simulink model "rccg_digitalTwin"  (R2024a)
settings: Solver=VariableStepAuto  StartTime=0.0  StopTime=1  RelTol=1e-3
libraries: spsMultimeterLib x14, spsThreePhaseBreakerLib x9, spsThreePhaseSeriesRLCLoadLib x7, spsThreePhaseVIMeasurementLib x3, spsSynchronousMachinepuStandardLib x2, spsThreePhaseTransformerTwoWindingsLib x1, spsExcitationSystemLib x1, spsHydraulicTurbineandGovernorLib x1, spsThreePhaseParallelRLCLoadLib x1, sps_lib x1
settings Model: Creator=dogba  LastModifiedBy=dogba

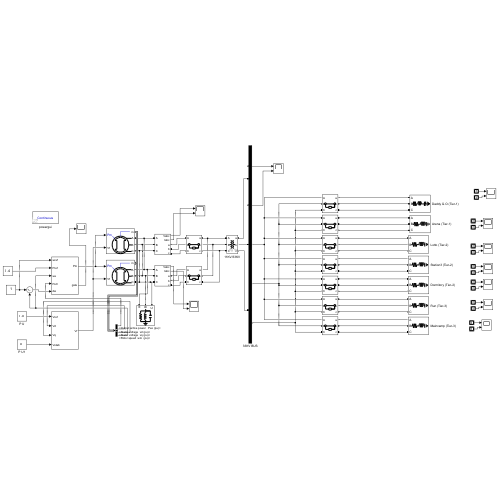
[thumbnail: Simulink's stored preview of the top-level diagram]
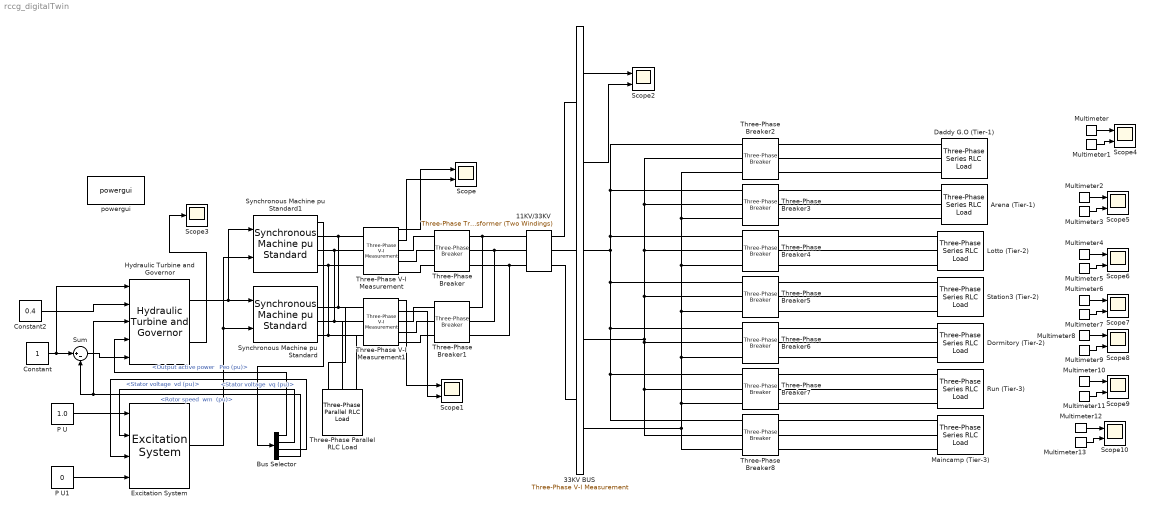
== system rccg_digitalTwin ==
  11KV/33KV : spsThreePhaseTransformerTwoWindingsLib/Three-Phase Transformer (Two Windings)  Winding1Connection=Yg  Winding2Connection=Yg  CoreType=Three single-phase transformers  SetSaturation=off  Hysteresis=off  DataFile='hysteresis'  SetInitialFlux=off  Measurements=None  UNITS=pu  NominalPower=[ 10e6 , 60 ]  Winding1=[ 11e3 , 0.002 , 0.08 ]  Winding2=[ 33e3 , 0.002 , 0.08 ]  Rm=500  Lm=500  L0=0.5  Saturation=[ 0,0 ; 0.0024,1.2 ; 1.0,1.52 ]  InitialFluxes=[ 0.8 , -0.8 , 0.7 ]  BreakLoop=off  DiscreteSolver=Trapezoidal iterative  DataType=off  TransfoNumber=1
  33KV BUS : spsThreePhaseVIMeasurementLib/Three-Phase V-I Measurement  VoltageMeasurement=phase-to-ground  SetLabelV=off  LabelV=Vabc  Vpu=off  VpuLL=off  CurrentMeasurement=yes  SetLabelI=off  LabelI=Iabc  Ipu=off  Pbase=100e6  Vbase=500e3  OutputType=Complex  PhasorSimulation=off  PSBequivalent=0
  Arena (Tier-1) : spsThreePhaseSeriesRLCLoadLib/Three-Phase Series RLC Load  LConnTagsString=A|B|C  Configuration=Y (grounded)  NominalVoltage=415  Vabc=[1e3 1e3 1e3]  Vabcp=[1e3 1e3 1e3]  NominalFrequency=50  UnbalancedPower=off  ActivePower=2e6  InductivePower=0.7e6  CapacitivePower=0  Pabc=[10e3 9e3 11e3]  QLabc=[100 90 110]  QCabc=[100 90 110]  Pabcp=[10e3 9e3 11e3]  QLabcp=[100 90 110]  QCabcp=[100 90 110]  Measurements=Branch voltages and currents  LoadType=constant PQ
  Bus Selector : BusSelector  OutputSignals="Output active power   Peo (pu),dq0 components.Stator voltage  vd (pu),dq0 components.Stator voltage  vq (pu),Mechanical.Rotor speed  wm  (pu)"
  Constant : Constant
  Constant2 : Constant  Value=0.4
  Daddy G.O (Tier-1) : spsThreePhaseSeriesRLCLoadLib/Three-Phase Series RLC Load  LConnTagsString=A|B|C  Configuration=Y (grounded)  NominalVoltage=415  Vabc=[1e3 1e3 1e3]  Vabcp=[1e3 1e3 1e3]  NominalFrequency=50  UnbalancedPower=off  ActivePower=1.5e6  InductivePower=0.4e6  CapacitivePower=100  Pabc=[10e3 9e3 11e3]  QLabc=[100 90 110]  QCabc=[100 90 110]  Pabcp=[10e3 9e3 11e3]  QLabcp=[100 90 110]  QCabcp=[100 90 110]  Measurements=Branch voltages and currents  LoadType=constant PQ
  Dormitory (Tier-2) : spsThreePhaseSeriesRLCLoadLib/Three-Phase Series RLC Load  LConnTagsString=A|B|C  Configuration=Y (grounded)  NominalVoltage=400  Vabc=[1e3 1e3 1e3]  Vabcp=[1e3 1e3 1e3]  NominalFrequency=50  UnbalancedPower=off  ActivePower=0.5e6  InductivePower=0.15e6  CapacitivePower=0  Pabc=[10e3 9e3 11e3]  QLabc=[100 90 110]  QCabc=[100 90 110]  Pabcp=[10e3 9e3 11e3]  QLabcp=[100 90 110]  QCabcp=[100 90 110]  Measurements=Branch voltages and currents  LoadType=constant PQ
  Excitation System : spsExcitationSystemLib/Excitation System  tr=20e-3  reg=[ 300, 0.001 ]  exc=[ 1, 0 ]  tgr=[ 0, 0 ]  damp=[ 0.001, 0.1 ]  sat=[ 0, 0 ]  lim=[ -11.5, 11.5, 0 ]  v0="[1.0  1.28]"
      settings: LibrarySourceBlock=sps_lib/Electrical Machines/Synchronous Machine Control/Excitation System
  Hydraulic Turbine and Governor : spsHydraulicTurbineandGovernorLib/Hydraulic Turbine and Governor  sm="[ 10/3  0.07 ]"  gate="[  0.01  0.97518  -0.1  0.1 ]"  reg="[  0.05  1.163  0.105  0  0.01  ]"  hyd="[  0  2.67  ]"  dref=0  po=0.7516
      settings: LibrarySourceBlock=|
      | sps_lib/Electrical Machines/Synchronous Machine Control/Hydraulic Turbine
      | and Governor
  Lotto (Tier-2) : spsThreePhaseSeriesRLCLoadLib/Three-Phase Series RLC Load  LConnTagsString=A|B|C  Configuration=Y (grounded)  NominalVoltage=415  Vabc=[1e3 1e3 1e3]  Vabcp=[1e3 1e3 1e3]  NominalFrequency=50  UnbalancedPower=off  ActivePower=0.8e6  InductivePower=0.2e6  CapacitivePower=0  Pabc=[10e3 9e3 11e3]  QLabc=[100 90 110]  QCabc=[100 90 110]  Pabcp=[10e3 9e3 11e3]  QLabcp=[100 90 110]  QCabcp=[100 90 110]  Measurements=Branch voltages and currents  LoadType=constant PQ
  Maincamp (Tier-3) : spsThreePhaseSeriesRLCLoadLib/Three-Phase Series RLC Load  LConnTagsString=A|B|C  Configuration=Y (grounded)  NominalVoltage=415  Vabc=[1e3 1e3 1e3]  Vabcp=[1e3 1e3 1e3]  NominalFrequency=50  UnbalancedPower=off  ActivePower=0.2e6  InductivePower=0.05e6  CapacitivePower=0  Pabc=[10e3 9e3 11e3]  QLabc=[100 90 110]  QCabc=[100 90 110]  Pabcp=[10e3 9e3 11e3]  QLabcp=[100 90 110]  QCabcp=[100 90 110]  Measurements=Branch voltages and currents  LoadType=constant PQ
  Multimeter : spsMultimeterLib/Multimeter  L=42  sel=[4 5 6]  yselected={}  Gain=[1 1 1]  OutputType=Complex  PlotAtSimulationStop=off  PhasorSimulation=off
  Multimeter1 : spsMultimeterLib/Multimeter  L=42  sel=[25 26 27]  yselected={}  Gain=[1 1 1]  OutputType=Complex  PlotAtSimulationStop=off  PhasorSimulation=off
  Multimeter10 : spsMultimeterLib/Multimeter  L=42  sel=[16 17 18]  yselected={}  Gain=[1 1 1]  OutputType=Complex  PlotAtSimulationStop=off  PhasorSimulation=off
  Multimeter11 : spsMultimeterLib/Multimeter  L=42  sel=[37 38 39]  yselected={}  Gain=[1 1 1]  OutputType=Complex  PlotAtSimulationStop=off  PhasorSimulation=off
  Multimeter12 : spsMultimeterLib/Multimeter  L=42  sel=[13 14 15]  yselected={}  Gain=[1 1 1]  OutputType=Complex  PlotAtSimulationStop=off  PhasorSimulation=off
  Multimeter13 : spsMultimeterLib/Multimeter  L=42  sel=[34 35 36]  yselected={}  Gain=[1 1 1]  OutputType=Complex  PlotAtSimulationStop=off  PhasorSimulation=off
  Multimeter2 : spsMultimeterLib/Multimeter  L=42  sel=[1 2 3]  yselected={}  Gain=[1 1 1]  OutputType=Complex  PlotAtSimulationStop=off  PhasorSimulation=off
  Multimeter3 : spsMultimeterLib/Multimeter  L=42  sel=[22 23 24]  yselected={}  Gain=[1 1 1]  OutputType=Complex  PlotAtSimulationStop=off  PhasorSimulation=off
  Multimeter4 : spsMultimeterLib/Multimeter  L=42  sel=[10 11 12]  yselected={}  Gain=[1 1 1]  OutputType=Complex  PlotAtSimulationStop=off  PhasorSimulation=off
  Multimeter5 : spsMultimeterLib/Multimeter  L=42  sel=[31 32 33]  yselected={}  Gain=[1 1 1]  OutputType=Complex  PlotAtSimulationStop=off  PhasorSimulation=off
  Multimeter6 : spsMultimeterLib/Multimeter  L=42  sel=[19 20 21]  yselected={}  Gain=[1 1 1]  OutputType=Complex  PlotAtSimulationStop=off  PhasorSimulation=off
  Multimeter7 : spsMultimeterLib/Multimeter  L=42  sel=[40 41 42]  yselected={}  Gain=[1 1 1]  OutputType=Complex  PlotAtSimulationStop=off  PhasorSimulation=off
  Multimeter8 : spsMultimeterLib/Multimeter  L=42  sel=[7 8 9]  yselected={}  Gain=[1 1 1]  OutputType=Complex  PlotAtSimulationStop=off  PhasorSimulation=off
  Multimeter9 : spsMultimeterLib/Multimeter  L=42  sel=[28 29 30]  yselected={}  Gain=[1 1 1]  OutputType=Complex  PlotAtSimulationStop=off  PhasorSimulation=off
  P U : Constant  Value=1.0
  P U1 : Constant  Value=0
  Run (Tier-3) : spsThreePhaseSeriesRLCLoadLib/Three-Phase Series RLC Load  LConnTagsString=A|B|C  Configuration=Y (grounded)  NominalVoltage=415  Vabc=[1e3 1e3 1e3]  Vabcp=[1e3 1e3 1e3]  NominalFrequency=50  UnbalancedPower=off  ActivePower=0.3e6  InductivePower=0.05e6  CapacitivePower=0  Pabc=[10e3 9e3 11e3]  QLabc=[100 90 110]  QCabc=[100 90 110]  Pabcp=[10e3 9e3 11e3]  QLabcp=[100 90 110]  QCabcp=[100 90 110]  Measurements=Branch voltages and currents  LoadType=constant PQ
  Scope{,1..2,4..10} (10 alike) : Scope  NumInputPorts=2
  Scope3 : Scope
  Station3 (Tier-2) : spsThreePhaseSeriesRLCLoadLib/Three-Phase Series RLC Load  LConnTagsString=A|B|C  Configuration=Y (grounded)  NominalVoltage=415  Vabc=[1e3 1e3 1e3]  Vabcp=[1e3 1e3 1e3]  NominalFrequency=50  UnbalancedPower=off  ActivePower=0.7e6  InductivePower=0.2e6  CapacitivePower=0  Pabc=[10e3 9e3 11e3]  QLabc=[100 90 110]  QCabc=[100 90 110]  Pabcp=[10e3 9e3 11e3]  QLabcp=[100 90 110]  QCabcp=[100 90 110]  Measurements=Branch voltages and currents  LoadType=constant Z
  Sum : Sum  Inputs=|+-
  Synchronous Machine pu Standard : spsSynchronousMachinepuStandardLib/Synchronous Machine pu Standard  PresetModel=No  MechanicalLoad=Mechanical power Pm  ShowDetailedParameters=on  RotorType=Salient-pole  Units=per unit standard parameters  MeasurementBus=off  NominalParameters=[5e6 11e3 50]  Reactances1=[ 1.81, 0.3, 0.23, 1.76, 0.65, 0.25, 0.15 ]  Reactances2=[2.24 0.17 0.12 1.02 0.13 0.08]  dAxisTimeConstants=Short-circuit  qAxisTimeConstants=Short-circuit  TimeConstants1="[ 4.4849  0.0681  0.1  ]"  TimeConstants2=[ 8.0, 0.03, 1.0, 0.07 ]  TimeConstants3="[  4.49  0.0681  0.0513  ]"  TimeConstants4=[ 8.0, 0.03, 0.3371, 0.0295 ]  TimeConstants5=[ 1.01, 0.053, 0.1 ]  TimeConstants6=[ 1.3201, 0.023, 1.0, 0.07 ]  TimeConstants7=[0.012 0.003 0.003]  TimeConstants8=[ 1.3201, 0.0231, 0.3371, 0.0295 ]  StatorResistance=0.037875  Mechanical=[0.1028 0.02056 2]  PolePairs=20  InitialConditions="[ 0  0  0  0  0  0  0  0  1 ]"  SetSaturation=on  Saturation=[0.6404,0.7127,0.8441,0.9214,0.9956,1.082,1.19,1.316,1.457;0.7,0.7698,0.8872,0.9466,0.9969,1.046,1.1,1.151,1.201]  LoadFlowParameters=[1,0,0,0,0]  TsPowergui=0  TsBlock=-1  IterativeModel=Trapezoidal non iterative  IterativeDiscreteModel=Trapezoidal non iterative  BusType=PV  Pref=0  Qref=0  Qmin=-inf  Qmax=inf  PLF=0  QLF=0
  Synchronous Machine pu Standard1 : spsSynchronousMachinepuStandardLib/Synchronous Machine pu Standard  PresetModel=No  MechanicalLoad=Mechanical power Pm  ShowDetailedParameters=on  RotorType=Salient-pole  Units=per unit standard parameters  MeasurementBus=off  NominalParameters=[5e6 11e3 50]  Reactances1=[ 1.81, 0.3, 0.23, 1.76, 0.65, 0.25, 0.15 ]  Reactances2=[2.24 0.17 0.12 1.02 0.13 0.08]  dAxisTimeConstants=Short-circuit  qAxisTimeConstants=Short-circuit  TimeConstants1="[ 4.4849  0.0681  0.1  ]"  TimeConstants2=[ 8.0, 0.03, 1.0, 0.07 ]  TimeConstants3="[  4.49  0.0681  0.0513  ]"  TimeConstants4=[ 8.0, 0.03, 0.3371, 0.0295 ]  TimeConstants5=[ 1.01, 0.053, 0.1 ]  TimeConstants6=[ 1.3201, 0.023, 1.0, 0.07 ]  TimeConstants7=[0.012 0.003 0.003]  TimeConstants8=[ 1.3201, 0.0231, 0.3371, 0.0295 ]  StatorResistance=0.037875  Mechanical=[0.1028 0.02056 2]  PolePairs=20  InitialConditions="[ 0  0  0  0  0  0  0  0  1 ]"  SetSaturation=on  Saturation=[0.6404,0.7127,0.8441,0.9214,0.9956,1.082,1.19,1.316,1.457;0.7,0.7698,0.8872,0.9466,0.9969,1.046,1.1,1.151,1.201]  LoadFlowParameters=[1,0,0,0,0]  TsPowergui=0  TsBlock=-1  IterativeModel=Trapezoidal non iterative  IterativeDiscreteModel=Trapezoidal non iterative  BusType=PV  Pref=0  Qref=0  Qmin=-inf  Qmax=inf  PLF=0  QLF=0
  Three-Phase Parallel RLC Load : spsThreePhaseParallelRLCLoadLib/Three-Phase Parallel RLC Load  LConnTagsString=A|B|C  Configuration=Y (grounded)  NominalVoltage=1000  Vabc=[1e3 1e3 1e3]  Vabcp=[1e3 1e3 1e3]  NominalFrequency=60  UnbalancedPower=off  ActivePower=10e3  InductivePower=100  CapacitivePower=100  Pabc=[10e3 9e3 11e3]  QLabc=[100 90 110]  QCabc=[100 90 110]  Pabcp=[10e3 9e3 11e3]  QLabcp=[100 90 110]  QCabcp=[100 90 110]  Measurements=None  LoadType=constant Z
  Three-Phase V-I Measurement : spsThreePhaseVIMeasurementLib/Three-Phase V-I Measurement  VoltageMeasurement=phase-to-ground  SetLabelV=off  LabelV=Vabc  Vpu=off  VpuLL=off  CurrentMeasurement=yes  SetLabelI=off  LabelI=Iabc  Ipu=off  Pbase=100e6  Vbase=500e3  OutputType=Complex  PhasorSimulation=off  PSBequivalent=0
  Three-Phase V-I Measurement1 : spsThreePhaseVIMeasurementLib/Three-Phase V-I Measurement  VoltageMeasurement=phase-to-ground  SetLabelV=off  LabelV=Vabc  Vpu=off  VpuLL=off  CurrentMeasurement=yes  SetLabelI=off  LabelI=Iabc  Ipu=off  Pbase=100e6  Vbase=500e3  OutputType=Complex  PhasorSimulation=off  PSBequivalent=0
  Three-Phase Breaker{,1..8} (9 alike) : spsThreePhaseBreakerLib/Three-Phase Breaker  InitialState=closed  SwitchA=on  SwitchB=on  SwitchC=on  SwitchTimes="[1/60  5/60]"  External=off  BreakerResistance=0.01  SnubberResistance=1e6  SnubberCapacitance=inf  Measurements=None
  powergui : sps_lib/powergui  Priority=1  SimulationMode=Continuous  SampleTime=50e-6  frequency=60  Iterations=50  frequencyindice=50  Pbase=100e6  ErrMax=1e-4  UnitsV=kV  UnitsW=MW  buscounter=0  FunctionMessages=off  echomessages=off  EnableUseOfTLC=off  CurrentSourceSwitches=off  DisableSnubberDevices=off  DisableRonSwitches=off  DisableVfSwitches=off  DisplayEquations=off  AutomaticDiscreteSolvers=off  SolverType=Tustin/Backward Euler (TBE)  Interpol=off  ExternalGateDelay=off  methode=off  Ts=100  x0status=blocks  SPID=on  SwTol=0  HookPort=off  NonlinearTolerance=1e-4  nMaxIteration=100  ContinueOnMaxIteration=off  RestoreLinks=warning  ResistiveCurrentMeasurement=off  Frange=[0:2:500]  Ylog=off  Xlog=on  ShowGrid=off  save=off  variable=ZData  structure=0  ZoomFFT=off  StartTime=0.0  cycles=1  DisplayStyle=1  fundamental=60  FreqAxis=off  MaxFrequency=1000  frequencyindicesteady=1  RmsSteady=1  display=off
  wires:
  Excitation System/1 -> Synchronous Machine pu Standard1/2, Synchronous Machine pu Standard/2
  Hydraulic Turbine and Governor/1 -> Synchronous Machine pu Standard1/1, Synchronous Machine pu Standard/1
  P U/1 -> Excitation System/1
  P U1/1 -> Excitation System/4
  Three-Phase V-I Measurement/1 -> Scope/1
  Three-Phase V-I Measurement/2 -> Scope/2
  Three-Phase V-I Measurement1/1 -> Scope1/1
  Three-Phase V-I Measurement1/2 -> Scope1/2
  Synchronous Machine pu Standard1/1 -> Bus Selector/1
  Bus Selector/1 -> Hydraulic Turbine and Governor/4  "<Output active power   Peo (pu)>"
  Bus Selector/2 -> Excitation System/2  "<Stator voltage  vd (pu)>"
  Bus Selector/3 -> Excitation System/3  "<Stator voltage  vq (pu)>"
  Bus Selector/4 -> Sum/2, Hydraulic Turbine and Governor/3  "<Rotor speed  wm  (pu)>"
  Constant/1 -> Hydraulic Turbine and Governor/1, Sum/1
  Sum/1 -> Hydraulic Turbine and Governor/5
  Constant2/1 -> Hydraulic Turbine and Governor/2
  33KV BUS/1 -> Scope2/1
  33KV BUS/2 -> Scope2/2
  Hydraulic Turbine and Governor/2 -> Scope3/1
  Multimeter/1 -> Scope4/1
  Multimeter1/1 -> Scope4/2
  Multimeter3/1 -> Scope5/2
  Multimeter2/1 -> Scope5/1
  Multimeter4/1 -> Scope6/1
  Multimeter5/1 -> Scope6/2
  Multimeter7/1 -> Scope7/2
  Multimeter6/1 -> Scope7/1
  Multimeter8/1 -> Scope8/1
  Multimeter9/1 -> Scope8/2
  Multimeter11/1 -> Scope9/2
  Multimeter10/1 -> Scope9/1
  Multimeter12/1 -> Scope10/1
  Multimeter13/1 -> Scope10/2
  connections:
  11KV/33KV/LConn1 -- Three-Phase Breaker1/RConn1 -- Three-Phase Breaker/RConn1
  11KV/33KV/LConn2 -- Three-Phase Breaker1/RConn2 -- Three-Phase Breaker/RConn2
  11KV/33KV/LConn3 -- Three-Phase Breaker1/RConn3 -- Three-Phase Breaker/RConn3
  33KV BUS/LConn2 -- 11KV/33KV/RConn2
  11KV/33KV/RConn1 -- 33KV BUS/LConn1
  11KV/33KV/RConn3 -- 33KV BUS/LConn3
  Three-Phase V-I Measurement/LConn1 -- Three-Phase Parallel RLC Load/LConn1 -- Three-Phase V-I Measurement1/LConn1 -- Synchronous Machine pu Standard/RConn1 -- Synchronous Machine pu Standard1/RConn1
  Three-Phase V-I Measurement/LConn2 -- Synchronous Machine pu Standard1/RConn2 -- Three-Phase Parallel RLC Load/LConn2 -- Three-Phase V-I Measurement1/LConn2 -- Synchronous Machine pu Standard/RConn2
  Three-Phase V-I Measurement/LConn3 -- Three-Phase Parallel RLC Load/LConn3 -- Three-Phase V-I Measurement1/LConn3 -- Synchronous Machine pu Standard/RConn3 -- Synchronous Machine pu Standard1/RConn3
  Three-Phase V-I Measurement1/RConn2 -- Three-Phase Breaker1/LConn2
  Three-Phase V-I Measurement1/RConn3 -- Three-Phase Breaker1/LConn3
  Three-Phase V-I Measurement1/RConn1 -- Three-Phase Breaker1/LConn1
  Three-Phase V-I Measurement/RConn3 -- Three-Phase Breaker/LConn3
  Three-Phase V-I Measurement/RConn2 -- Three-Phase Breaker/LConn2
  Three-Phase V-I Measurement/RConn1 -- Three-Phase Breaker/LConn1
  Three-Phase Breaker2/RConn2 -- Daddy G.O (Tier-1)/LConn2
  Three-Phase Breaker2/RConn1 -- Daddy G.O (Tier-1)/LConn1
  Three-Phase Breaker2/RConn3 -- Daddy G.O (Tier-1)/LConn3
  Three-Phase Breaker8/RConn1 -- Maincamp (Tier-3)/LConn1
  Three-Phase Breaker8/RConn2 -- Maincamp (Tier-3)/LConn2
  Three-Phase Breaker8/RConn3 -- Maincamp (Tier-3)/LConn3
  Three-Phase Breaker7/RConn3 -- Run (Tier-3)/LConn3
  Three-Phase Breaker7/RConn2 -- Run (Tier-3)/LConn2
  Three-Phase Breaker7/RConn1 -- Run (Tier-3)/LConn1
  Three-Phase Breaker6/RConn3 -- Dormitory (Tier-2)/LConn3
  Three-Phase Breaker6/RConn2 -- Dormitory (Tier-2)/LConn2
  Three-Phase Breaker6/RConn1 -- Dormitory (Tier-2)/LConn1
  Three-Phase Breaker5/RConn3 -- Station3 (Tier-2)/LConn3
  Three-Phase Breaker5/RConn2 -- Station3 (Tier-2)/LConn2
  Three-Phase Breaker5/RConn1 -- Station3 (Tier-2)/LConn1
  Three-Phase Breaker4/RConn3 -- Lotto (Tier-2)/LConn3
  Three-Phase Breaker4/RConn2 -- Lotto (Tier-2)/LConn2
  Three-Phase Breaker4/RConn1 -- Lotto (Tier-2)/LConn1
  Three-Phase Breaker3/RConn3 -- Arena (Tier-1)/LConn3
  Three-Phase Breaker3/RConn2 -- Arena (Tier-1)/LConn2
  Three-Phase Breaker3/RConn1 -- Arena (Tier-1)/LConn1
  Three-Phase Breaker8/LConn1 -- Three-Phase Breaker7/LConn1 -- Three-Phase Breaker6/LConn1 -- Three-Phase Breaker5/LConn1 -- 33KV BUS/RConn1 -- Three-Phase Breaker4/LConn1 -- Three-Phase Breaker3/LConn1 -- Three-Phase Breaker2/LConn1
  Three-Phase Breaker2/LConn2 -- Three-Phase Breaker3/LConn2 -- Three-Phase Breaker4/LConn2 -- Three-Phase Breaker5/LConn2 -- 33KV BUS/RConn2 -- Three-Phase Breaker6/LConn2 -- Three-Phase Breaker7/LConn2 -- Three-Phase Breaker8/LConn2
  Three-Phase Breaker2/LConn3 -- Three-Phase Breaker3/LConn3 -- Three-Phase Breaker8/LConn3 -- 33KV BUS/RConn3 -- Three-Phase Breaker7/LConn3 -- Three-Phase Breaker6/LConn3 -- Three-Phase Breaker5/LConn3 -- Three-Phase Breaker4/LConn3
